simulink model "tiltrotor_model6"  (R2023a)
settings: Solver=VariableStepAuto  StartTime=0.0  StopTime=30  RelTol=1e-3
values from neighbouring files (symbols this model uses):
  g = 9.81    [LQR_controller_pitching.m]    (also in MPC_controller_pitching.m; MPC_vs_LQR.m; simulation_parameters.m)
  G = zeros(n*(N+1), m*N)    [MPC_vs_LQR.m]
  H = zeros(n*(N+1), n)    [MPC_vs_LQR.m]    (also in Schur_solver.m = [A, -B*(R\B'))
  I = diag([0.018 0.035 0.051])    [simulation_parameters.m]
  initial = [0 0 0 0 0 0]'    [simulation_parameters.m]
  kf = 65    [simulation_parameters.m]
  Lh = 0.2    [simulation_parameters.m]
  Lv = 0.2    [simulation_parameters.m]
  m = 1.12    [LQR_controller_pitching.m]    (also in MPC_vs_LQR.m = size(Bd,2); simulation_parameters.m)
  N = 150    [MPC_controller_pitching.m]    (also in MPC_vs_LQR.m = 20)
  p_D = 0    [controller_parameters_model_5_and_6.m]
  p_I = 0    [controller_parameters_model_5_and_6.m]
  p_P = 0.35    [controller_parameters_model_5_and_6.m]
  pitch_D = 0.4    [controller_parameters.m]    (also in controller_parameters_model_3_and_4.m; controller_parameters_model_5_and_6.m = 0)
  pitch_I = 0    [controller_parameters.m]    (also in controller_parameters_model_3_and_4.m; controller_parameters_model_5_and_6.m)
  pitch_P = 1.4    [controller_parameters.m]    (also in controller_parameters_model_3_and_4.m; controller_parameters_model_5_and_6.m = 10)
  Q1 = diag(ones(n*(N+1),1)) * Q1_0    [MPC_vs_LQR.m]
  Q2 = diag(ones(m*N,1)) * Q2_0    [MPC_vs_LQR.m]
  r_D = 0    [controller_parameters_model_5_and_6.m]
  r_I = 0    [controller_parameters_model_5_and_6.m]
  r_P = 1    [controller_parameters_model_5_and_6.m]
  reference = [1 1 1 0 40 50]'    [simulation_parameters.m]
  roll_D = 0.3    [controller_parameters.m]    (also in controller_parameters_model_3_and_4.m; controller_parameters_model_5_and_6.m = 1)
  roll_I = 0    [controller_parameters.m]    (also in controller_parameters_model_3_and_4.m; controller_parameters_model_5_and_6.m)
  roll_P = 1.5    [controller_parameters.m]    (also in controller_parameters_model_3_and_4.m; controller_parameters_model_5_and_6.m = 8)
  s_r = [1 1 1 1 1 1]    [simulation_parameters.m]
  Tmax = 4    [simulation_parameters.m]
  toll = 1e-12    [simulation_parameters.m]
  vy_D = 0    [controller_parameters.m]    (also in controller_parameters_model_3_and_4.m; controller_parameters_model_5_and_6.m)
  vy_I = 0    [controller_parameters.m]    (also in controller_parameters_model_3_and_4.m; controller_parameters_model_5_and_6.m)
  vy_P = 5    [controller_parameters.m]    (also in controller_parameters_model_3_and_4.m; controller_parameters_model_5_and_6.m = 12)
  x_D = 0.7    [controller_parameters.m]    (also in controller_parameters_model_3_and_4.m; controller_parameters_model_5_and_6.m = 0)
  x_I = 0    [controller_parameters.m]    (also in controller_parameters_model_3_and_4.m; controller_parameters_model_5_and_6.m)
  x_P = 1.8    [controller_parameters.m]    (also in controller_parameters_model_3_and_4.m; controller_parameters_model_5_and_6.m = 1.5)
  y_D = 0.7    [controller_parameters.m]    (also in controller_parameters_model_3_and_4.m; controller_parameters_model_5_and_6.m = 0.3)
  y_I = 0    [controller_parameters.m]    (also in controller_parameters_model_3_and_4.m; controller_parameters_model_5_and_6.m)
  y_P = 1.8    [controller_parameters.m]    (also in controller_parameters_model_3_and_4.m; controller_parameters_model_5_and_6.m = 1.5)
  yaw_D = 0.5    [controller_parameters.m]    (also in controller_parameters_model_3_and_4.m = 0.3; controller_parameters_model_5_and_6.m = 0)
  yaw_I = 0    [controller_parameters.m]    (also in controller_parameters_model_3_and_4.m; controller_parameters_model_5_and_6.m)
  yaw_P = 1    [controller_parameters.m]    (also in controller_parameters_model_3_and_4.m; controller_parameters_model_5_and_6.m = 1.5)
  z_D = 0    [controller_parameters.m]    (also in controller_parameters_model_3_and_4.m; controller_parameters_model_5_and_6.m)
  z_I = 0    [controller_parameters.m]    (also in controller_parameters_model_3_and_4.m; controller_parameters_model_5_and_6.m)
  z_P = 3    [controller_parameters.m]    (also in controller_parameters_model_3_and_4.m; controller_parameters_model_5_and_6.m = 2.5)
libraries: slpidlib x10, simulink x6, simulink_extras x1, mpclib x1, matrix_library x1
(part 2 of 2)

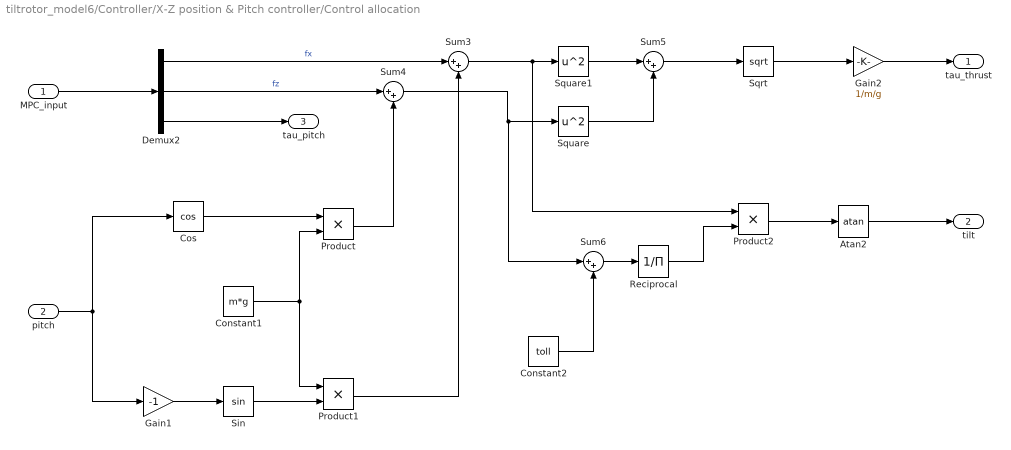
== system tiltrotor_model6/Controller/X-Z position & Pitch controller/Control allocation ==
  MPC_input : Inport
  pitch : Inport  Port=2
  Atan2 : Trigonometry  Operator=atan
  Constant1 : Constant  Value=m*g
  Constant2 : Constant  Value=toll
  Cos : Trigonometry  Operator=cos
  Demux2 : Demux  Outputs=3
  Gain1 : Gain  Gain=-1
  Gain2 : Gain  Gain=1/m/g
  Product : Product
  Product1 : Product
  Product2 : Product
  Reciprocal : Product  Inputs=/
  Sin : Trigonometry
  Sqrt : Sqrt
  Square : Math  Operator=square
  Square1 : Math  Operator=square
  Sum{3..6} (4 alike) : Sum  Inputs=|++
  tau_thrust : Outport
  tilt : Outport  Port=2
  tau_pitch : Outport  Port=3
  wires:
  Square1/1 -> Sum5/1
  pitch/1 -> Gain1/1, Cos/1
  Atan2/1 -> tilt/1
  Product1/1 -> Sum3/2
  Sin/1 -> Product1/2
  Sum6/1 -> Reciprocal/1
  Sum5/1 -> Sqrt/1
  Sqrt/1 -> Gain2/1
  Gain2/1 -> tau_thrust/1
  Product/1 -> Sum4/2
  Square/1 -> Sum5/2
  Cos/1 -> Product/1
  Sum3/1 -> Product2/1, Square1/1
  Constant2/1 -> Sum6/2
  Demux2/1 -> Sum3/1  "fx"
  Demux2/2 -> Sum4/1  "fz"
  Gain1/1 -> Sin/1
  Constant1/1 -> Product/2, Product1/1
  Reciprocal/1 -> Product2/2
  Sum4/1 -> Sum6/1, Square/1
  Demux2/3 -> tau_pitch/1
  MPC_input/1 -> Demux2/1
  Product2/1 -> Atan2/1

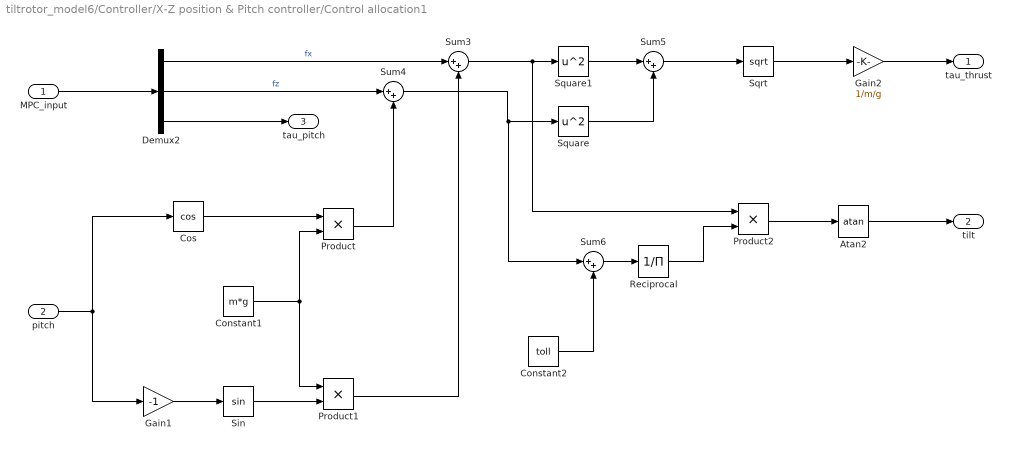
== system tiltrotor_model6/Controller/X-Z position & Pitch controller/Control allocation1 ==
  MPC_input : Inport
  pitch : Inport  Port=2
  Atan2 : Trigonometry  Operator=atan
  Constant1 : Constant  Value=m*g
  Constant2 : Constant  Value=toll
  Cos : Trigonometry  Operator=cos
  Demux2 : Demux  Outputs=3
  Gain1 : Gain  Gain=-1
  Gain2 : Gain  Gain=1/m/g
  Product : Product
  Product1 : Product
  Product2 : Product
  Reciprocal : Product  Inputs=/
  Sin : Trigonometry
  Sqrt : Sqrt
  Square : Math  Operator=square
  Square1 : Math  Operator=square
  Sum{3..6} (4 alike) : Sum  Inputs=|++
  tau_thrust : Outport
  tilt : Outport  Port=2
  tau_pitch : Outport  Port=3
  wires:
  Square1/1 -> Sum5/1
  pitch/1 -> Gain1/1, Cos/1
  Atan2/1 -> tilt/1
  Product1/1 -> Sum3/2
  Sin/1 -> Product1/2
  Sum6/1 -> Reciprocal/1
  Sum5/1 -> Sqrt/1
  Sqrt/1 -> Gain2/1
  Gain2/1 -> tau_thrust/1
  Product/1 -> Sum4/2
  Square/1 -> Sum5/2
  Cos/1 -> Product/1
  Sum3/1 -> Product2/1, Square1/1
  Constant2/1 -> Sum6/2
  Demux2/1 -> Sum3/1  "fx"
  Demux2/2 -> Sum4/1  "fz"
  Gain1/1 -> Sin/1
  Constant1/1 -> Product/2, Product1/1
  Reciprocal/1 -> Product2/2
  Sum4/1 -> Sum6/1, Square/1
  Demux2/3 -> tau_pitch/1
  MPC_input/1 -> Demux2/1
  Product2/1 -> Atan2/1

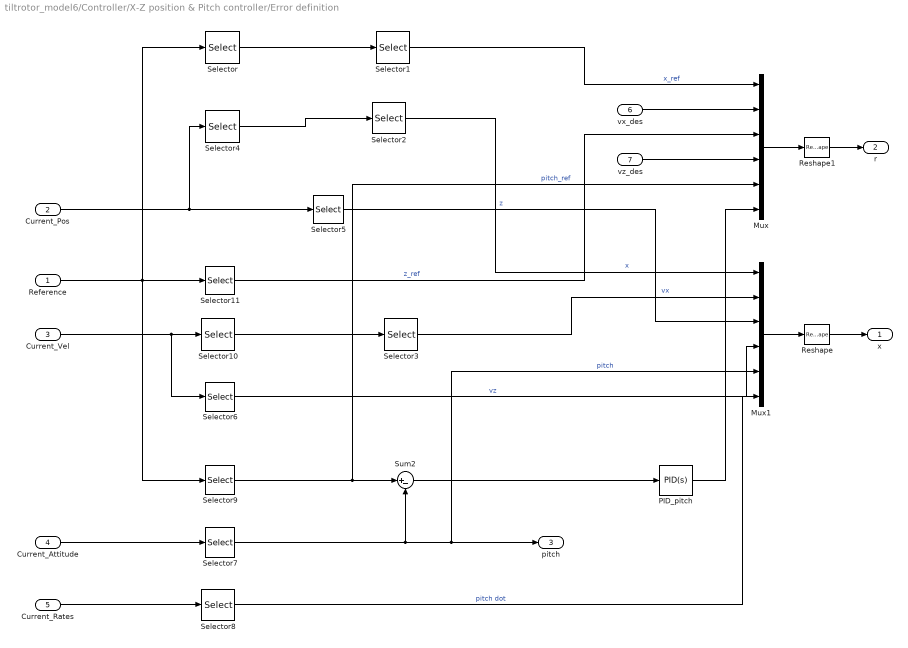
== system tiltrotor_model6/Controller/X-Z position & Pitch controller/Error definition ==
  Reference : Inport
  Current_Pos : Inport  Port=2
  Current_Vel : Inport  Port=3
  Current_Attitude : Inport  Port=4
  Current_Rates : Inport  Port=5
  vx_des : Inport  Port=6
  vz_des : Inport  Port=7
  Mux : Mux  Inputs=6
  Mux1 : Mux  Inputs=6
  PID_pitch : slpidlib/PID Controller  Controller=PID  Form=Parallel  TimeDomain=Continuous-time  UseExternalTs=off  SampleTime=-1  IntegratorMethod=Forward Euler  FilterMethod=Forward Euler  ControllerParametersSource=internal  P=pitch_P  I=pitch_I  UseKiTs=off  D=pitch_D  N=100  UseFilter=on  TunerSelectOption=Transfer Function Based (PID Tuner App)  InitialConditionSource=internal  InitialConditionForIntegrator=0  InitialConditionForFilter=0  DifferentiatorICPrevScaledInput=0  ExternalReset=none  TrackingMode=off  Kt=1  LimitOutput=off  SatLimitsSource=internal  UpperSaturationLimit=inf  LowerSaturationLimit=-inf  LinearizeAsGain=on  AntiWindupMode=none  Kb=1  LimitIntegrator=off  UpperIntegratorSaturationLimit=inf  LowerIntegratorSaturationLimit=-inf  POutMin=[]  POutMax=[]  IOutMin=[]  IOutMax=[]  DOutMin=[]  DOutMax=[]  NOutMin=[]  NOutMax=[]  SumOutMin=[]  SumOutMax=[]  SaturationOutMin=[]  SaturationOutMax=[]  PParamMin=[]  PParamMax=[]  IParamMin=[]  IParamMax=[]  DParamMin=[]  DParamMax=[]  NParamMin=[]  NParamMax=[]  KbParamMin=[]  KbParamMax=[]  KtParamMin=[]  KtParamMax=[]  KbOutMin=[]  KbOutMax=[]  KtOutMin=[]  KtOutMax=[]  IntegratorOutMin=[]  IntegratorOutMax=[]  FilterOutMin=[]  FilterOutMax=[]  SumI1OutMin=[]  SumI1OutMax=[]  SumI2OutMin=[]  SumI2OutMax=[]  SumI3OutMin=[]  SumI3OutMax=[]  SumI4OutMin=[]  SumI4OutMax=[]  SumDOutMin=[]  SumDOutMax=[]  DifferentiatorOutMin=[]  DifferentiatorOutMax=[]  FilterDiffOutCoefMin=[]  FilterDiffOutCoefMax=[]  ReciprocalOutMin=[]  ReciprocalOutMax=[]  SumDenOutMin=[]  SumDenOutMax=[]  SumNumOutMin=[]  SumNumOutMax=[]  DivideOutMin=[]  DivideOutMax=[]  UdiffTsProdOutMin=[]  UdiffTsProdOutMax=[]  NTsProdOutMin=[]  NTsProdOutMax=[]  UintegralTsProdOutMin=[]  UintegralTsProdOutMax=[]  UngainTsProdOutMin=[]  UngainTsProdOutMax=[]  ClampingZeroOutDataTypeStr=Inherit: Inherit via back propagation  ClampingZeroOutMin=[]  ClampingZeroOutMax=[]  FilterDenConstantOutDataTypeStr=Inherit: Inherit via back propagation  FilterDenConstantOutMin=[]  FilterDenConstantOutMax=[]  PCopyOutDataTypeStr=Inherit: Inherit via back propagation  PCopyOutMin=[]  PCopyOutMax=[]  NCopyOutDataTypeStr=Inherit: Inherit via back propagation  NCopyOutMin=[]  NCopyOutMax=[]  IntegratorContinuousStateAttributes=''  IntegratorStateMustResolveToSignalObject=off  IntegratorRTWStateStorageClass=Auto  FilterContinuousStateAttributes=''  FilterStateMustResolveToSignalObject=off  FilterRTWStateStorageClass=Auto  ParallelPVariant=InternalParameters  IdealPVariant=Disabled  IVariant=InternalParameters  DVariant=InternalParameters  IntegratorVariant=Continuous  SatVariant=Disabled  AWVariant=Passthrough  PCopyVariant=Disabled  TRVariant=Disabled  FdbkBlocksVariant=Forward  IdealPFdbkVariant=Disabled  SatFdbkVariant=Disabled  DerivativeFilterVariant=ContFilter  NVariant=InternalParameters  NCopyVariant=Disabled  FilterICVariant=InternalICsFilter  IntegratorICVariant=InternalICs  ExternalResetVariant=Disabled  TRSumVariant=Passthrough  SumFdbkVariant=Disabled  SumVariant=Sum_PID  TsampFilterVariant=InternalTs  TsampNgainVariant=Passthrough  TsampIntegralVariant=Disabled_SignalSpec  ExternalSaturationOutDataTypeStr=Inherit: Same as second input
  Reshape : Reshape  OutputDimensionality=Column vector (2-D)
  Reshape1 : Reshape  OutputDimensionality=Column vector (2-D)
  Selector : Selector  InputPortWidth=6  IndexOptions=Index vector (dialog)  Indices=[1 2]  OutputSizes=1
  Selector1 : Selector  InputPortWidth=2  IndexOptions=Index vector (dialog)  Indices=[1]  OutputSizes=1
  Selector10 : Selector  InputPortWidth=3  IndexOptions=Index vector (dialog)  Indices=[1 2]  OutputSizes=1
  Selector11 : Selector  InputPortWidth=6  IndexOptions=Index vector (dialog)  Indices=[3]  OutputSizes=1
  Selector2 : Selector  InputPortWidth=2  IndexOptions=Index vector (dialog)  Indices=[1]  OutputSizes=1
  Selector3 : Selector  InputPortWidth=2  IndexOptions=Index vector (dialog)  Indices=[1]  OutputSizes=1
  Selector4 : Selector  InputPortWidth=3  IndexOptions=Index vector (dialog)  Indices=[1 2]  OutputSizes=1
  Selector5 : Selector  InputPortWidth=3  IndexOptions=Index vector (dialog)  Indices=[3]  OutputSizes=1
  Selector6 : Selector  InputPortWidth=3  IndexOptions=Index vector (dialog)  Indices=[3]  OutputSizes=1
  Selector7 : Selector  InputPortWidth=3  IndexOptions=Index vector (dialog)  Indices=[2]  OutputSizes=1
  Selector8 : Selector  InputPortWidth=3  IndexOptions=Index vector (dialog)  Indices=[2]  OutputSizes=1
  Selector9 : Selector  InputPortWidth=6  IndexOptions=Index vector (dialog)  Indices=[5]  OutputSizes=1
  Sum2 : Sum  Inputs=|+-
  x : Outport
  r : Outport  Port=2
  pitch : Outport  Port=3
  wires:
  Selector10/1 -> Selector3/1
  Current_Rates/1 -> Selector8/1
  Sum2/1 -> PID_pitch/1
  Current_Attitude/1 -> Selector7/1
  Selector9/1 -> Mux/5, Sum2/1  "pitch_ref"
  Reference/1 -> Selector/1, Selector11/1, Selector9/1
  Current_Vel/1 -> Selector10/1, Selector6/1
  Selector7/1 -> Mux1/5, pitch/1, Sum2/2  "pitch"
  Selector/1 -> Selector1/1
  Current_Pos/1 -> Selector5/1, Selector4/1
  Selector1/1 -> Mux/1  "x_ref"
  Selector11/1 -> Mux/3  "z_ref"
  vx_des/1 -> Mux/2
  vz_des/1 -> Mux/4
  PID_pitch/1 -> Mux/6
  Selector2/1 -> Mux1/1  "x"
  Selector3/1 -> Mux1/2  "vx"
  Selector6/1 -> Mux1/4  "vz"
  Selector5/1 -> Mux1/3  "z"
  Selector8/1 -> Mux1/6  "pitch dot"
  Mux/1 -> Reshape1/1
  Mux1/1 -> Reshape/1
  Reshape/1 -> x/1
  Reshape1/1 -> r/1
  Selector4/1 -> Selector2/1

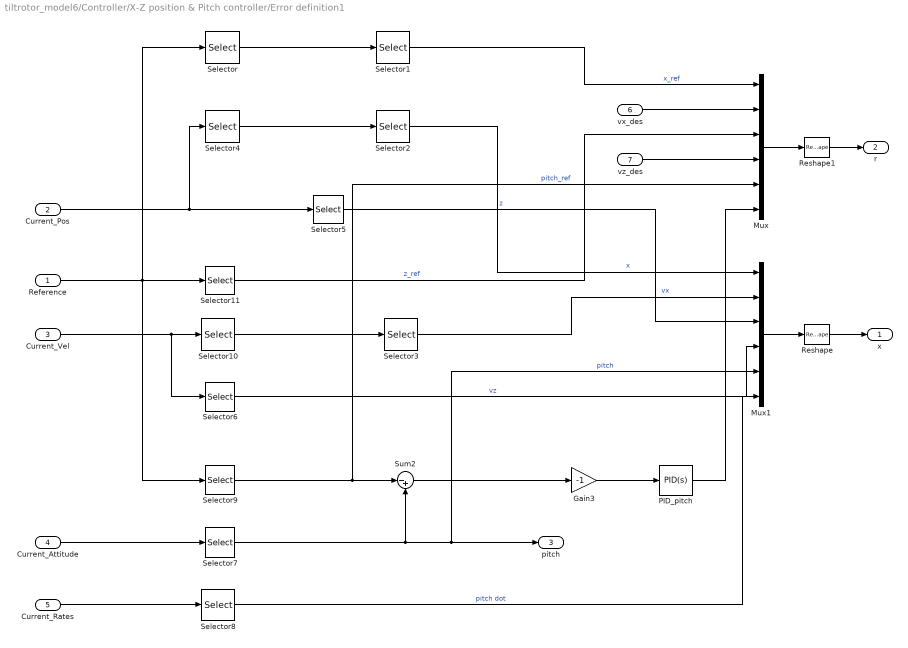
== system tiltrotor_model6/Controller/X-Z position & Pitch controller/Error definition1 ==
  Reference : Inport
  Current_Pos : Inport  Port=2
  Current_Vel : Inport  Port=3
  Current_Attitude : Inport  Port=4
  Current_Rates : Inport  Port=5
  vx_des : Inport  Port=6
  vz_des : Inport  Port=7
  Gain3 : Gain  Gain=-1
  Mux : Mux  Inputs=6
  Mux1 : Mux  Inputs=6
  PID_pitch : slpidlib/PID Controller  Controller=PID  Form=Parallel  TimeDomain=Continuous-time  UseExternalTs=off  SampleTime=-1  IntegratorMethod=Forward Euler  FilterMethod=Forward Euler  ControllerParametersSource=internal  P=pitch_P  I=pitch_I  UseKiTs=off  D=pitch_D  N=100  UseFilter=on  TunerSelectOption=Transfer Function Based (PID Tuner App)  InitialConditionSource=internal  InitialConditionForIntegrator=0  InitialConditionForFilter=0  DifferentiatorICPrevScaledInput=0  ExternalReset=none  TrackingMode=off  Kt=1  LimitOutput=off  SatLimitsSource=internal  UpperSaturationLimit=inf  LowerSaturationLimit=-inf  LinearizeAsGain=on  AntiWindupMode=none  Kb=1  LimitIntegrator=off  UpperIntegratorSaturationLimit=inf  LowerIntegratorSaturationLimit=-inf  POutMin=[]  POutMax=[]  IOutMin=[]  IOutMax=[]  DOutMin=[]  DOutMax=[]  NOutMin=[]  NOutMax=[]  SumOutMin=[]  SumOutMax=[]  SaturationOutMin=[]  SaturationOutMax=[]  PParamMin=[]  PParamMax=[]  IParamMin=[]  IParamMax=[]  DParamMin=[]  DParamMax=[]  NParamMin=[]  NParamMax=[]  KbParamMin=[]  KbParamMax=[]  KtParamMin=[]  KtParamMax=[]  KbOutMin=[]  KbOutMax=[]  KtOutMin=[]  KtOutMax=[]  IntegratorOutMin=[]  IntegratorOutMax=[]  FilterOutMin=[]  FilterOutMax=[]  SumI1OutMin=[]  SumI1OutMax=[]  SumI2OutMin=[]  SumI2OutMax=[]  SumI3OutMin=[]  SumI3OutMax=[]  SumI4OutMin=[]  SumI4OutMax=[]  SumDOutMin=[]  SumDOutMax=[]  DifferentiatorOutMin=[]  DifferentiatorOutMax=[]  FilterDiffOutCoefMin=[]  FilterDiffOutCoefMax=[]  ReciprocalOutMin=[]  ReciprocalOutMax=[]  SumDenOutMin=[]  SumDenOutMax=[]  SumNumOutMin=[]  SumNumOutMax=[]  DivideOutMin=[]  DivideOutMax=[]  UdiffTsProdOutMin=[]  UdiffTsProdOutMax=[]  NTsProdOutMin=[]  NTsProdOutMax=[]  UintegralTsProdOutMin=[]  UintegralTsProdOutMax=[]  UngainTsProdOutMin=[]  UngainTsProdOutMax=[]  ClampingZeroOutDataTypeStr=Inherit: Inherit via back propagation  ClampingZeroOutMin=[]  ClampingZeroOutMax=[]  FilterDenConstantOutDataTypeStr=Inherit: Inherit via back propagation  FilterDenConstantOutMin=[]  FilterDenConstantOutMax=[]  PCopyOutDataTypeStr=Inherit: Inherit via back propagation  PCopyOutMin=[]  PCopyOutMax=[]  NCopyOutDataTypeStr=Inherit: Inherit via back propagation  NCopyOutMin=[]  NCopyOutMax=[]  IntegratorContinuousStateAttributes=''  IntegratorStateMustResolveToSignalObject=off  IntegratorRTWStateStorageClass=Auto  FilterContinuousStateAttributes=''  FilterStateMustResolveToSignalObject=off  FilterRTWStateStorageClass=Auto  ParallelPVariant=InternalParameters  IdealPVariant=Disabled  IVariant=InternalParameters  DVariant=InternalParameters  IntegratorVariant=Continuous  SatVariant=Disabled  AWVariant=Passthrough  PCopyVariant=Disabled  TRVariant=Disabled  FdbkBlocksVariant=Forward  IdealPFdbkVariant=Disabled  SatFdbkVariant=Disabled  DerivativeFilterVariant=ContFilter  NVariant=InternalParameters  NCopyVariant=Disabled  FilterICVariant=InternalICsFilter  IntegratorICVariant=InternalICs  ExternalResetVariant=Disabled  TRSumVariant=Passthrough  SumFdbkVariant=Disabled  SumVariant=Sum_PID  TsampFilterVariant=InternalTs  TsampNgainVariant=Passthrough  TsampIntegralVariant=Disabled_SignalSpec  ExternalSaturationOutDataTypeStr=Inherit: Same as second input
  Reshape : Reshape  OutputDimensionality=Column vector (2-D)
  Reshape1 : Reshape  OutputDimensionality=Column vector (2-D)
  Selector : Selector  InputPortWidth=6  IndexOptions=Index vector (dialog)  Indices=[1 2]  OutputSizes=1
  Selector1 : Selector  InputPortWidth=2  IndexOptions=Index vector (dialog)  Indices=[1]  OutputSizes=1
  Selector10 : Selector  InputPortWidth=3  IndexOptions=Index vector (dialog)  Indices=[1 2]  OutputSizes=1
  Selector11 : Selector  InputPortWidth=6  IndexOptions=Index vector (dialog)  Indices=[3]  OutputSizes=1
  Selector2 : Selector  InputPortWidth=2  IndexOptions=Index vector (dialog)  Indices=[1]  OutputSizes=1
  Selector3 : Selector  InputPortWidth=2  IndexOptions=Index vector (dialog)  Indices=[1]  OutputSizes=1
  Selector4 : Selector  InputPortWidth=3  IndexOptions=Index vector (dialog)  Indices=[1 2]  OutputSizes=1
  Selector5 : Selector  InputPortWidth=3  IndexOptions=Index vector (dialog)  Indices=[3]  OutputSizes=1
  Selector6 : Selector  InputPortWidth=3  IndexOptions=Index vector (dialog)  Indices=[3]  OutputSizes=1
  Selector7 : Selector  InputPortWidth=3  IndexOptions=Index vector (dialog)  Indices=[2]  OutputSizes=1
  Selector8 : Selector  InputPortWidth=3  IndexOptions=Index vector (dialog)  Indices=[2]  OutputSizes=1
  Selector9 : Selector  InputPortWidth=6  IndexOptions=Index vector (dialog)  Indices=[5]  OutputSizes=1
  Sum2 : Sum  Inputs=|-+
  x : Outport
  r : Outport  Port=2
  pitch : Outport  Port=3
  wires:
  Sum2/1 -> Gain3/1
  Selector10/1 -> Selector3/1
  Current_Rates/1 -> Selector8/1
  Gain3/1 -> PID_pitch/1
  Current_Attitude/1 -> Selector7/1
  Selector9/1 -> Mux/5, Sum2/1  "pitch_ref"
  Reference/1 -> Selector/1, Selector11/1, Selector9/1
  Current_Vel/1 -> Selector10/1, Selector6/1
  Selector7/1 -> Mux1/5, pitch/1, Sum2/2  "pitch"
  Selector/1 -> Selector1/1
  Current_Pos/1 -> Selector5/1, Selector4/1
  Selector4/1 -> Selector2/1
  Selector1/1 -> Mux/1  "x_ref"
  Selector11/1 -> Mux/3  "z_ref"
  vx_des/1 -> Mux/2
  vz_des/1 -> Mux/4
  PID_pitch/1 -> Mux/6
  Selector2/1 -> Mux1/1  "x"
  Selector3/1 -> Mux1/2  "vx"
  Selector6/1 -> Mux1/4  "vz"
  Selector5/1 -> Mux1/3  "z"
  Selector8/1 -> Mux1/6  "pitch dot"
  Mux/1 -> Reshape1/1
  Mux1/1 -> Reshape/1
  Reshape/1 -> x/1
  Reshape1/1 -> r/1

== matlab function tiltrotor_model6/Controller/X-Z position & Pitch controller/MATLAB Function1 ==
  data: r input; MPC_input output; x input; G input; H input; Q1 input; Q2 input; N input
function MPC_input = fcn(r, x, G, H, Q1, Q2, N)

r = repmat(r, N+1, 1);

% Compute cost function
P_lq = G' * Q1 * G + Q2;
q_lq = (H*x - r)' * Q1 * G;

% Solve (no constraints)
U_opt = -P_lq \ q_lq';
MPC_input = U_opt(1:3);

== matlab function tiltrotor_model6/Control allocation/MATLAB Function ==
  data: tilt input; C output; Lh input; Lv input; kf input
function C = fcn(tilt, Lh, Lv, kf)

s = sin(tilt);
c = cos(tilt);
kf = 1/kf;

C = [ s,  s,  s,  s;
      c,  c,  c,  c;
    -Lh*c - kf*s,  Lh*c + kf*s,  Lh*c - kf*s,  -Lh*c + kf*s;
    -Lv*c, -Lv*c,  Lv*c,  Lv*c;
     Lh*s - kf*c, -Lh*s + kf*c, -Lh*s - kf*c,  Lh*s + kf*c ];

== matlab function tiltrotor_model6/UAV/Rotation mat  ==
  data: psi input; R output
function R = get_r_mat(psi)
%
% inertial to body frame
%
R = [cos(psi) -sin(psi); sin(psi) cos(psi)]';

== matlab function tiltrotor_model6/Control allocation/MATLAB Function1 ==
  data: eta input; D output; Lv input; Lh input; kf input
function D = fcn(eta, Lv, Lh, kf)

kf = 1/kf;

D = 0.25*[1, -1/kf * sin(eta) - 1/Lh * cos(eta), - 1/Lv / cos(eta), -1/kf * cos(eta) + 1/Lh * sin(eta);
    1, 1/kf * sin(eta) + 1/Lh * cos(eta), - 1/Lv / cos(eta), 1/kf * cos(eta) - 1/Lh * sin(eta);
    1, -1/kf * sin(eta) + 1/Lh * cos(eta), 1/Lv / cos(eta), -1/kf * cos(eta) - 1/Lh * sin(eta);
    1, 1/kf * sin(eta) - 1/Lh * cos(eta), 1/Lv / cos(eta), 1/kf * cos(eta) + 1/Lh * sin(eta)];

== matlab function tiltrotor_model6/UAV/Dynamics of phi/MATLAB Function1 ==
  data: phi input; Q output
function Q = fcn(phi)

roll = phi(1);
pitch = phi(2);

Q = euler_to_body_angvel(roll, pitch);

== matlab function tiltrotor_model6/UAV/MATLAB Function ==
  data: Rx output; Ry output; Rz output; phi input
function [Rx, Ry, Rz]  = fcn(phi)

roll = phi(1);
pitch = phi(2);
yaw = phi(3);

[Rx, Ry, Rz] = rotation_matrices(roll, pitch, yaw);
